simulink model "controlador_automatico_osc"  (R2023b)
settings: Solver=VariableStepAuto  StartTime=0.0  StopTime=10.0  RelTol=1e-3
undefined symbols (not defined in the file): g, m_t
settings Model: Creator=renzo  LastModifiedBy=renzo

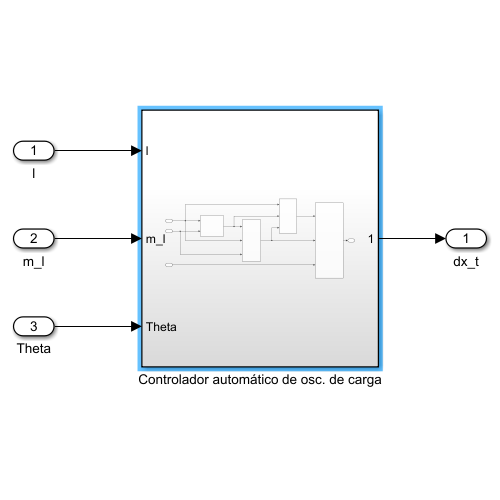
[thumbnail: Simulink's stored preview of the top-level diagram]
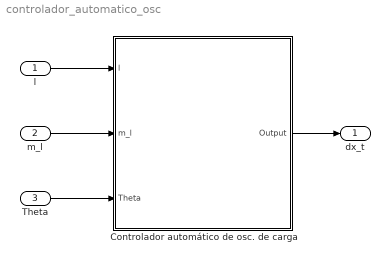
== system controlador_automatico_osc ==
  l : Inport
  m_l : Inport  Port=2
  Theta : Inport  Port=3
  Controlador automático de osc. de carga : Subsystem
  dx_t : Outport
  wires:
  l/1 -> Controlador automático de osc. de carga/1(l)
  m_l/1 -> Controlador automático de osc. de carga/2(m_l)
  Theta/1 -> Controlador automático de osc. de carga/3(Theta)
  Controlador automático de osc. de carga/1(Output) -> dx_t/1

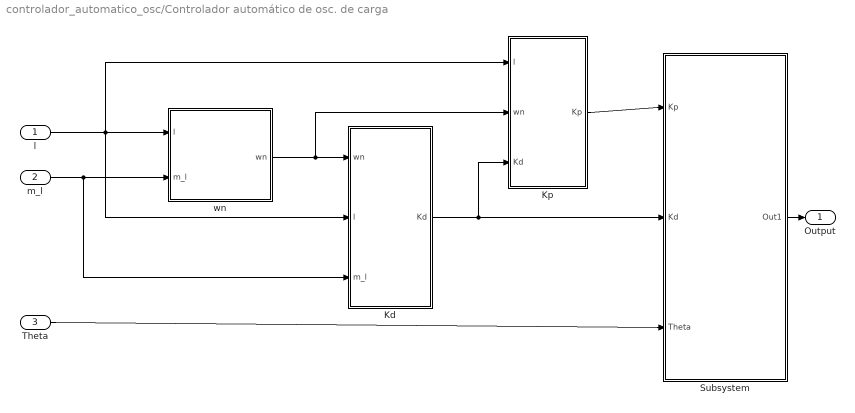
== system controlador_automatico_osc/Controlador automático de osc. de carga ==
  l : Inport
  m_l : Inport  Port=2
  Theta : Inport  Port=3
  Kd : Subsystem
  Kp : Subsystem
  Subsystem : Subsystem
  wn : Subsystem
  Output : Outport
  wires:
  wn/1(wn) -> Kp/2(wn), Kd/1(wn)
  Kd/1(Kd) -> Kp/3(Kd), Subsystem/2(Kd)
  m_l/1 -> wn/2(m_l), Kd/3(m_l)
  Theta/1 -> Subsystem/3(Theta)
  l/1 -> Kp/1(l), Kd/2(l), wn/1(l)
  Kp/1(Kp) -> Subsystem/1(Kp)
  Subsystem/1(Out1) -> Output/1

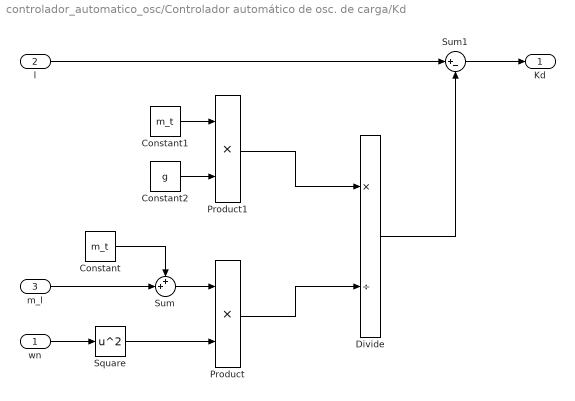
== system controlador_automatico_osc/Controlador automático de osc. de carga/Kd ==
  wn : Inport
  l : Inport  Port=2
  m_l : Inport  Port=3
  Constant : Constant  Value=m_t
  Constant1 : Constant  Value=m_t
  Constant2 : Constant  Value=g
  Divide : Product  Inputs=*/
  Product : Product
  Product1 : Product
  Square : Math  Operator=square
  Sum : Sum  Inputs=++|
  Sum1 : Sum  Inputs=|+-
  Kd : Outport
  wires:
  m_l/1 -> Sum/2
  Constant/1 -> Sum/1
  wn/1 -> Square/1
  Square/1 -> Product/2
  Sum/1 -> Product/1
  Constant2/1 -> Product1/2
  Constant1/1 -> Product1/1
  Product1/1 -> Divide/1
  Product/1 -> Divide/2
  Divide/1 -> Sum1/2
  Sum1/1 -> Kd/1
  l/1 -> Sum1/1

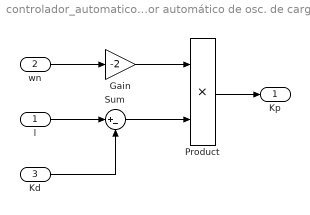
== system controlador_automatico_osc/Controlador automático de osc. de carga/Kp ==
  l : Inport
  wn : Inport  Port=2
  Kd : Inport  Port=3
  Gain : Gain  Gain=-2
  Product : Product
  Sum : Sum  Inputs=|+-
  Kp : Outport
  wires:
  wn/1 -> Gain/1
  Gain/1 -> Product/1
  l/1 -> Sum/1
  Kd/1 -> Sum/2
  Sum/1 -> Product/2
  Product/1 -> Kp/1

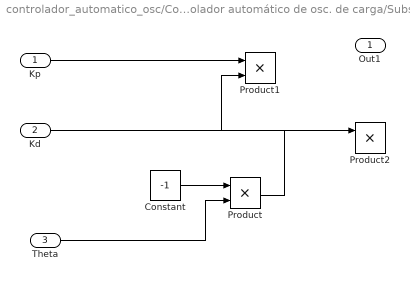
== system controlador_automatico_osc/Controlador automático de osc. de carga/Subsystem ==
  Kp : Inport
  Kd : Inport  Port=2
  Theta : Inport  Port=3
  Constant : Constant  Value=-1
  Product : Product
  Product1 : Product
  Product2 : Product
  Out1 : Outport
  wires:
  Constant/1 -> Product/1
  Theta/1 -> Product/2
  Kp/1 -> Product1/1
  Product/1 -> Product1/2
  Kd/1 -> Product2/1

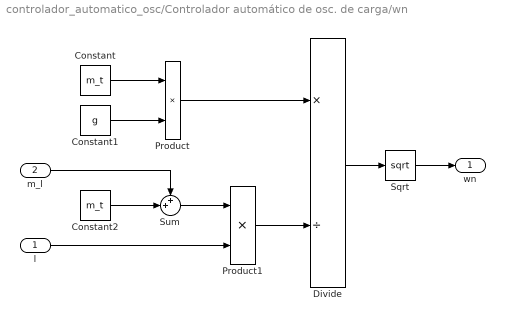
== system controlador_automatico_osc/Controlador automático de osc. de carga/wn ==
  l : Inport
  m_l : Inport  Port=2
  Constant : Constant  Value=m_t
  Constant1 : Constant  Value=g
  Constant2 : Constant  Value=m_t
  Divide : Product  Inputs=*/
  Product : Product
  Product1 : Product
  Sqrt : Sqrt
  Sum : Sum  Inputs=++|
  wn : Outport
  wires:
  Constant/1 -> Product/1
  Constant1/1 -> Product/2
  Product/1 -> Divide/1
  Sum/1 -> Product1/1
  l/1 -> Product1/2
  Product1/1 -> Divide/2
  Divide/1 -> Sqrt/1
  Sqrt/1 -> wn/1
  Constant2/1 -> Sum/2
  m_l/1 -> Sum/1
